simulink model "LM_TOS_0120"  (R2018b)
settings: Solver=FixedStepDiscrete  StartTime=0.0  StopTime=inf  FixedStep=0.005  RelTol=1e-3
PostLoadFcn:
  | if any(exist('dsrtsu_mdlpostloadfcn', 'file') ~= 0), dsrtsu_mdlpostloadfcn('Execute', bdroot); end
libraries: rtican x35
(part 9 of 11)

== system LM_TOS_0120/LM_TOS_MODEL/adapter2/hmi_output_adapter ==
  In1 : Inport  OutDataTypeStr=Bus: HMI_OUTPUT_ST_APT
  Bus Creator : BusCreator  Inputs=1  OutDataTypeStr=Bus: HMI_DISPLAY_ARRAY_ST  NonVirtualBus=on
  Bus Selector1 : BusSelector  OutputSignals=obj_0,obj_1,obj_2,obj_3,obj_4,obj_5,obj_6,obj_7,obj_8,obj_9,obj_10,obj_11,obj_12,obj_13,obj_14,obj_15,obj_16,obj_17,obj_18,obj_19,obj_20,obj_21,obj_22,obj_23,obj_24,obj_25,obj_26,obj_27,obj_28,obj_29,obj_30,obj_31
  Vector Concatenate : Concatenate  NumInputs=32
  Out1 : Outport  OutDataTypeStr=Bus: HMI_DISPLAY_ARRAY_ST
  wires:
  Vector Concatenate/1 -> Bus Creator/1
  In1/1 -> Bus Selector1/1
  Bus Creator/1 -> Out1/1
  Bus Selector1/9 -> Vector Concatenate/9  "<obj_8>"
  Bus Selector1/1 -> Vector Concatenate/1  "<obj_0>"
  Bus Selector1/2 -> Vector Concatenate/2  "<obj_1>"
  Bus Selector1/3 -> Vector Concatenate/3  "<obj_2>"
  Bus Selector1/4 -> Vector Concatenate/4  "<obj_3>"
  Bus Selector1/5 -> Vector Concatenate/5  "<obj_4>"
  Bus Selector1/6 -> Vector Concatenate/6  "<obj_5>"
  Bus Selector1/7 -> Vector Concatenate/7  "<obj_6>"
  Bus Selector1/8 -> Vector Concatenate/8  "<obj_7>"
  Bus Selector1/10 -> Vector Concatenate/10  "<obj_9>"
  Bus Selector1/11 -> Vector Concatenate/11  "<obj_10>"
  Bus Selector1/12 -> Vector Concatenate/12  "<obj_11>"
  Bus Selector1/13 -> Vector Concatenate/13  "<obj_12>"
  Bus Selector1/14 -> Vector Concatenate/14  "<obj_13>"
  Bus Selector1/15 -> Vector Concatenate/15  "<obj_14>"
  Bus Selector1/16 -> Vector Concatenate/16  "<obj_15>"
  Bus Selector1/17 -> Vector Concatenate/17  "<obj_16>"
  Bus Selector1/18 -> Vector Concatenate/18  "<obj_17>"
  Bus Selector1/19 -> Vector Concatenate/19  "<obj_18>"
  Bus Selector1/20 -> Vector Concatenate/20  "<obj_19>"
  Bus Selector1/21 -> Vector Concatenate/21  "<obj_20>"
  Bus Selector1/22 -> Vector Concatenate/22  "<obj_21>"
  Bus Selector1/23 -> Vector Concatenate/23  "<obj_22>"
  Bus Selector1/24 -> Vector Concatenate/24  "<obj_23>"
  Bus Selector1/25 -> Vector Concatenate/25  "<obj_24>"
  Bus Selector1/26 -> Vector Concatenate/26  "<obj_25>"
  Bus Selector1/27 -> Vector Concatenate/27  "<obj_26>"
  Bus Selector1/28 -> Vector Concatenate/28  "<obj_27>"
  Bus Selector1/29 -> Vector Concatenate/29  "<obj_28>"
  Bus Selector1/30 -> Vector Concatenate/30  "<obj_29>"
  Bus Selector1/31 -> Vector Concatenate/31  "<obj_30>"
  Bus Selector1/32 -> Vector Concatenate/32  "<obj_31>"

== system LM_TOS_0120/RTI Data/RTI Data Store/RTI Data Store ==
  RTI Data Store : Subsystem  mask(RTI_DATA_STORE){}
      mask help:
      | RTI Data Store Block. This block is used by RTI to store internal model dependent data. Deleting this block will result in data loss.
      |
      | NEVER DELETE, COPY, OR MODIFY THIS BLOCK!
      mask Help:
      | RTI Data Store Block. This block is used by RTI to store internal model dependent data. Deleting this block will result in data loss.
      | 
      | NEVER DELETE, COPY, OR MODIFY THIS BLOCK!
      mask Display: text(0.5, 0.5, ' ', 'HorizontalAlignment', 'center');

== system LM_TOS_0120/LM_TOS_MODEL/adapter2/HWA_TAR_OBJ_ADP/Subsystem0 ==
  <target_object_adapter> : Inport
  Bus Creator1 : BusCreator  Inputs=9  OutDataTypeStr=Bus: TARGETOBJECT  NonVirtualBus=on
  Bus Selector4 : BusSelector  OutputSignals=dis2EgoLaneCenter,TTC_f,ID_un8,Index_un8,probWithinLane_arr_f_0,probWithinLane_arr_f_1,probWithinLane_arr_f_2,probWithinLane_arr_f_3,probWithinLane_arr_f_4,probCutIn_f,probCutOut_f,overlap_f,trackingTimeWithinLane_f
  Vector Concatenate : Concatenate  NumInputs=5
  TARGRTOBJECTS_ST : Outport  OutDataTypeStr=Bus: TARGETOBJECT
  wires:
  Bus Selector4/8 -> Vector Concatenate/4  "<probWithinLane_arr_f_3>"
  Bus Selector4/11 -> Bus Creator1/7  "<probCutOut_f>"
  Bus Selector4/10 -> Bus Creator1/6  "<probCutIn_f>"
  Bus Selector4/12 -> Bus Creator1/8  "<overlap_f>"
  Bus Selector4/9 -> Vector Concatenate/5  "<probWithinLane_arr_f_4>"
  Bus Selector4/2 -> Bus Creator1/2  "<TTC_f>"
  Bus Selector4/5 -> Vector Concatenate/1  "<probWithinLane_arr_f_0>"
  <target_object_adapter>/1 -> Bus Selector4/1
  Bus Selector4/6 -> Vector Concatenate/2  "<probWithinLane_arr_f_1>"
  Bus Selector4/13 -> Bus Creator1/9  "<trackingTimeWithinLane_f>"
  Bus Selector4/1 -> Bus Creator1/1  "<dis2EgoLaneCenter>"
  Bus Selector4/7 -> Vector Concatenate/3  "<probWithinLane_arr_f_2>"
  Vector Concatenate/1 -> Bus Creator1/5
  Bus Selector4/3 -> Bus Creator1/3  "<ID_un8>"
  Bus Creator1/1 -> TARGRTOBJECTS_ST/1
  Bus Selector4/4 -> Bus Creator1/4  "<Index_un8>"

== system LM_TOS_0120/LM_TOS_MODEL/adapter2/HWA_TAR_OBJ_ADP/Subsystem1 ==
  <target_object_adapter> : Inport
  Bus Creator1 : BusCreator  Inputs=9  OutDataTypeStr=Bus: TARGETOBJECT  NonVirtualBus=on
  Bus Selector4 : BusSelector  OutputSignals=dis2EgoLaneCenter,TTC_f,ID_un8,Index_un8,probWithinLane_arr_f_0,probWithinLane_arr_f_1,probWithinLane_arr_f_2,probWithinLane_arr_f_3,probWithinLane_arr_f_4,probCutIn_f,probCutOut_f,overlap_f,trackingTimeWithinLane_f
  Vector Concatenate : Concatenate  NumInputs=5
  TARGRTOBJECTS_ST : Outport  OutDataTypeStr=Bus: TARGETOBJECT
  wires:
  Bus Selector4/4 -> Bus Creator1/4  "<Index_un8>"
  Bus Creator1/1 -> TARGRTOBJECTS_ST/1
  Bus Selector4/3 -> Bus Creator1/3  "<ID_un8>"
  Vector Concatenate/1 -> Bus Creator1/5
  Bus Selector4/7 -> Vector Concatenate/3  "<probWithinLane_arr_f_2>"
  Bus Selector4/1 -> Bus Creator1/1  "<dis2EgoLaneCenter>"
  Bus Selector4/13 -> Bus Creator1/9  "<trackingTimeWithinLane_f>"
  Bus Selector4/6 -> Vector Concatenate/2  "<probWithinLane_arr_f_1>"
  <target_object_adapter>/1 -> Bus Selector4/1
  Bus Selector4/5 -> Vector Concatenate/1  "<probWithinLane_arr_f_0>"
  Bus Selector4/2 -> Bus Creator1/2  "<TTC_f>"
  Bus Selector4/9 -> Vector Concatenate/5  "<probWithinLane_arr_f_4>"
  Bus Selector4/12 -> Bus Creator1/8  "<overlap_f>"
  Bus Selector4/10 -> Bus Creator1/6  "<probCutIn_f>"
  Bus Selector4/11 -> Bus Creator1/7  "<probCutOut_f>"
  Bus Selector4/8 -> Vector Concatenate/4  "<probWithinLane_arr_f_3>"

== system LM_TOS_0120/LM_TOS_MODEL/adapter2/HWA_TAR_OBJ_ADP/Subsystem10 ==
  <target_object_adapter> : Inport
  Bus Creator1 : BusCreator  Inputs=9  OutDataTypeStr=Bus: TARGETOBJECT  NonVirtualBus=on
  Bus Selector4 : BusSelector  OutputSignals=dis2EgoLaneCenter,TTC_f,ID_un8,Index_un8,probWithinLane_arr_f_0,probWithinLane_arr_f_1,probWithinLane_arr_f_2,probWithinLane_arr_f_3,probWithinLane_arr_f_4,probCutIn_f,probCutOut_f,overlap_f,trackingTimeWithinLane_f
  Vector Concatenate : Concatenate  NumInputs=5
  TARGRTOBJECTS_ST : Outport  OutDataTypeStr=Bus: TARGETOBJECT
  wires:
  Bus Selector4/8 -> Vector Concatenate/4  "<probWithinLane_arr_f_3>"
  Bus Selector4/11 -> Bus Creator1/7  "<probCutOut_f>"
  Bus Selector4/10 -> Bus Creator1/6  "<probCutIn_f>"
  Bus Selector4/12 -> Bus Creator1/8  "<overlap_f>"
  Bus Selector4/9 -> Vector Concatenate/5  "<probWithinLane_arr_f_4>"
  Bus Selector4/2 -> Bus Creator1/2  "<TTC_f>"
  Bus Selector4/5 -> Vector Concatenate/1  "<probWithinLane_arr_f_0>"
  <target_object_adapter>/1 -> Bus Selector4/1
  Bus Selector4/6 -> Vector Concatenate/2  "<probWithinLane_arr_f_1>"
  Bus Selector4/13 -> Bus Creator1/9  "<trackingTimeWithinLane_f>"
  Bus Selector4/1 -> Bus Creator1/1  "<dis2EgoLaneCenter>"
  Bus Selector4/7 -> Vector Concatenate/3  "<probWithinLane_arr_f_2>"
  Vector Concatenate/1 -> Bus Creator1/5
  Bus Selector4/3 -> Bus Creator1/3  "<ID_un8>"
  Bus Creator1/1 -> TARGRTOBJECTS_ST/1
  Bus Selector4/4 -> Bus Creator1/4  "<Index_un8>"

== system LM_TOS_0120/LM_TOS_MODEL/adapter2/HWA_TAR_OBJ_ADP/Subsystem11 ==
  <target_object_adapter> : Inport
  Bus Creator1 : BusCreator  Inputs=9  OutDataTypeStr=Bus: TARGETOBJECT  NonVirtualBus=on
  Bus Selector4 : BusSelector  OutputSignals=dis2EgoLaneCenter,TTC_f,ID_un8,Index_un8,probWithinLane_arr_f_0,probWithinLane_arr_f_1,probWithinLane_arr_f_2,probWithinLane_arr_f_3,probWithinLane_arr_f_4,probCutIn_f,probCutOut_f,overlap_f,trackingTimeWithinLane_f
  Vector Concatenate : Concatenate  NumInputs=5
  TARGRTOBJECTS_ST : Outport  OutDataTypeStr=Bus: TARGETOBJECT
  wires:
  Bus Selector4/4 -> Bus Creator1/4  "<Index_un8>"
  Bus Creator1/1 -> TARGRTOBJECTS_ST/1
  Bus Selector4/3 -> Bus Creator1/3  "<ID_un8>"
  Vector Concatenate/1 -> Bus Creator1/5
  Bus Selector4/7 -> Vector Concatenate/3  "<probWithinLane_arr_f_2>"
  Bus Selector4/1 -> Bus Creator1/1  "<dis2EgoLaneCenter>"
  Bus Selector4/13 -> Bus Creator1/9  "<trackingTimeWithinLane_f>"
  Bus Selector4/6 -> Vector Concatenate/2  "<probWithinLane_arr_f_1>"
  <target_object_adapter>/1 -> Bus Selector4/1
  Bus Selector4/5 -> Vector Concatenate/1  "<probWithinLane_arr_f_0>"
  Bus Selector4/2 -> Bus Creator1/2  "<TTC_f>"
  Bus Selector4/9 -> Vector Concatenate/5  "<probWithinLane_arr_f_4>"
  Bus Selector4/12 -> Bus Creator1/8  "<overlap_f>"
  Bus Selector4/10 -> Bus Creator1/6  "<probCutIn_f>"
  Bus Selector4/11 -> Bus Creator1/7  "<probCutOut_f>"
  Bus Selector4/8 -> Vector Concatenate/4  "<probWithinLane_arr_f_3>"

== system LM_TOS_0120/LM_TOS_MODEL/adapter2/HWA_TAR_OBJ_ADP/Subsystem2 ==
  <target_object_adapter> : Inport
  Bus Creator1 : BusCreator  Inputs=9  OutDataTypeStr=Bus: TARGETOBJECT  NonVirtualBus=on
  Bus Selector4 : BusSelector  OutputSignals=dis2EgoLaneCenter,TTC_f,ID_un8,Index_un8,probWithinLane_arr_f_0,probWithinLane_arr_f_1,probWithinLane_arr_f_2,probWithinLane_arr_f_3,probWithinLane_arr_f_4,probCutIn_f,probCutOut_f,overlap_f,trackingTimeWithinLane_f
  Vector Concatenate : Concatenate  NumInputs=5
  TARGRTOBJECTS_ST : Outport  OutDataTypeStr=Bus: TARGETOBJECT
  wires:
  Bus Selector4/8 -> Vector Concatenate/4  "<probWithinLane_arr_f_3>"
  Bus Selector4/11 -> Bus Creator1/7  "<probCutOut_f>"
  Bus Selector4/10 -> Bus Creator1/6  "<probCutIn_f>"
  Bus Selector4/12 -> Bus Creator1/8  "<overlap_f>"
  Bus Selector4/9 -> Vector Concatenate/5  "<probWithinLane_arr_f_4>"
  Bus Selector4/2 -> Bus Creator1/2  "<TTC_f>"
  Bus Selector4/5 -> Vector Concatenate/1  "<probWithinLane_arr_f_0>"
  <target_object_adapter>/1 -> Bus Selector4/1
  Bus Selector4/6 -> Vector Concatenate/2  "<probWithinLane_arr_f_1>"
  Bus Selector4/13 -> Bus Creator1/9  "<trackingTimeWithinLane_f>"
  Bus Selector4/1 -> Bus Creator1/1  "<dis2EgoLaneCenter>"
  Bus Selector4/7 -> Vector Concatenate/3  "<probWithinLane_arr_f_2>"
  Vector Concatenate/1 -> Bus Creator1/5
  Bus Selector4/3 -> Bus Creator1/3  "<ID_un8>"
  Bus Creator1/1 -> TARGRTOBJECTS_ST/1
  Bus Selector4/4 -> Bus Creator1/4  "<Index_un8>"

== system LM_TOS_0120/LM_TOS_MODEL/adapter2/HWA_TAR_OBJ_ADP/Subsystem3 ==
  <target_object_adapter> : Inport
  Bus Creator1 : BusCreator  Inputs=9  OutDataTypeStr=Bus: TARGETOBJECT  NonVirtualBus=on
  Bus Selector4 : BusSelector  OutputSignals=dis2EgoLaneCenter,TTC_f,ID_un8,Index_un8,probWithinLane_arr_f_0,probWithinLane_arr_f_1,probWithinLane_arr_f_2,probWithinLane_arr_f_3,probWithinLane_arr_f_4,probCutIn_f,probCutOut_f,overlap_f,trackingTimeWithinLane_f
  Vector Concatenate : Concatenate  NumInputs=5
  TARGRTOBJECTS_ST : Outport  OutDataTypeStr=Bus: TARGETOBJECT
  wires:
  Bus Selector4/4 -> Bus Creator1/4  "<Index_un8>"
  Bus Creator1/1 -> TARGRTOBJECTS_ST/1
  Bus Selector4/3 -> Bus Creator1/3  "<ID_un8>"
  Vector Concatenate/1 -> Bus Creator1/5
  Bus Selector4/7 -> Vector Concatenate/3  "<probWithinLane_arr_f_2>"
  Bus Selector4/1 -> Bus Creator1/1  "<dis2EgoLaneCenter>"
  Bus Selector4/13 -> Bus Creator1/9  "<trackingTimeWithinLane_f>"
  Bus Selector4/6 -> Vector Concatenate/2  "<probWithinLane_arr_f_1>"
  <target_object_adapter>/1 -> Bus Selector4/1
  Bus Selector4/5 -> Vector Concatenate/1  "<probWithinLane_arr_f_0>"
  Bus Selector4/2 -> Bus Creator1/2  "<TTC_f>"
  Bus Selector4/9 -> Vector Concatenate/5  "<probWithinLane_arr_f_4>"
  Bus Selector4/12 -> Bus Creator1/8  "<overlap_f>"
  Bus Selector4/10 -> Bus Creator1/6  "<probCutIn_f>"
  Bus Selector4/11 -> Bus Creator1/7  "<probCutOut_f>"
  Bus Selector4/8 -> Vector Concatenate/4  "<probWithinLane_arr_f_3>"

== system LM_TOS_0120/LM_TOS_MODEL/adapter2/HWA_TAR_OBJ_ADP/Subsystem4 ==
  <target_object_adapter> : Inport
  Bus Creator1 : BusCreator  Inputs=9  OutDataTypeStr=Bus: TARGETOBJECT  NonVirtualBus=on
  Bus Selector4 : BusSelector  OutputSignals=dis2EgoLaneCenter,TTC_f,ID_un8,Index_un8,probWithinLane_arr_f_0,probWithinLane_arr_f_1,probWithinLane_arr_f_2,probWithinLane_arr_f_3,probWithinLane_arr_f_4,probCutIn_f,probCutOut_f,overlap_f,trackingTimeWithinLane_f
  Vector Concatenate : Concatenate  NumInputs=5
  TARGRTOBJECTS_ST : Outport  OutDataTypeStr=Bus: TARGETOBJECT
  wires:
  Bus Selector4/8 -> Vector Concatenate/4  "<probWithinLane_arr_f_3>"
  Bus Selector4/11 -> Bus Creator1/7  "<probCutOut_f>"
  Bus Selector4/10 -> Bus Creator1/6  "<probCutIn_f>"
  Bus Selector4/12 -> Bus Creator1/8  "<overlap_f>"
  Bus Selector4/9 -> Vector Concatenate/5  "<probWithinLane_arr_f_4>"
  Bus Selector4/2 -> Bus Creator1/2  "<TTC_f>"
  Bus Selector4/5 -> Vector Concatenate/1  "<probWithinLane_arr_f_0>"
  <target_object_adapter>/1 -> Bus Selector4/1
  Bus Selector4/6 -> Vector Concatenate/2  "<probWithinLane_arr_f_1>"
  Bus Selector4/13 -> Bus Creator1/9  "<trackingTimeWithinLane_f>"
  Bus Selector4/1 -> Bus Creator1/1  "<dis2EgoLaneCenter>"
  Bus Selector4/7 -> Vector Concatenate/3  "<probWithinLane_arr_f_2>"
  Vector Concatenate/1 -> Bus Creator1/5
  Bus Selector4/3 -> Bus Creator1/3  "<ID_un8>"
  Bus Creator1/1 -> TARGRTOBJECTS_ST/1
  Bus Selector4/4 -> Bus Creator1/4  "<Index_un8>"

== system LM_TOS_0120/LM_TOS_MODEL/adapter2/HWA_TAR_OBJ_ADP/Subsystem5 ==
  <target_object_adapter> : Inport
  Bus Creator1 : BusCreator  Inputs=9  OutDataTypeStr=Bus: TARGETOBJECT  NonVirtualBus=on
  Bus Selector4 : BusSelector  OutputSignals=dis2EgoLaneCenter,TTC_f,ID_un8,Index_un8,probWithinLane_arr_f_0,probWithinLane_arr_f_1,probWithinLane_arr_f_2,probWithinLane_arr_f_3,probWithinLane_arr_f_4,probCutIn_f,probCutOut_f,overlap_f,trackingTimeWithinLane_f
  Vector Concatenate : Concatenate  NumInputs=5
  TARGRTOBJECTS_ST : Outport  OutDataTypeStr=Bus: TARGETOBJECT
  wires:
  Bus Selector4/4 -> Bus Creator1/4  "<Index_un8>"
  Bus Creator1/1 -> TARGRTOBJECTS_ST/1
  Bus Selector4/3 -> Bus Creator1/3  "<ID_un8>"
  Vector Concatenate/1 -> Bus Creator1/5
  Bus Selector4/7 -> Vector Concatenate/3  "<probWithinLane_arr_f_2>"
  Bus Selector4/1 -> Bus Creator1/1  "<dis2EgoLaneCenter>"
  Bus Selector4/13 -> Bus Creator1/9  "<trackingTimeWithinLane_f>"
  Bus Selector4/6 -> Vector Concatenate/2  "<probWithinLane_arr_f_1>"
  <target_object_adapter>/1 -> Bus Selector4/1
  Bus Selector4/5 -> Vector Concatenate/1  "<probWithinLane_arr_f_0>"
  Bus Selector4/2 -> Bus Creator1/2  "<TTC_f>"
  Bus Selector4/9 -> Vector Concatenate/5  "<probWithinLane_arr_f_4>"
  Bus Selector4/12 -> Bus Creator1/8  "<overlap_f>"
  Bus Selector4/10 -> Bus Creator1/6  "<probCutIn_f>"
  Bus Selector4/11 -> Bus Creator1/7  "<probCutOut_f>"
  Bus Selector4/8 -> Vector Concatenate/4  "<probWithinLane_arr_f_3>"

== system LM_TOS_0120/LM_TOS_MODEL/adapter2/HWA_TAR_OBJ_ADP/Subsystem6 ==
  <target_object_adapter> : Inport
  Bus Creator1 : BusCreator  Inputs=9  OutDataTypeStr=Bus: TARGETOBJECT  NonVirtualBus=on
  Bus Selector4 : BusSelector  OutputSignals=dis2EgoLaneCenter,TTC_f,ID_un8,Index_un8,probWithinLane_arr_f_0,probWithinLane_arr_f_1,probWithinLane_arr_f_2,probWithinLane_arr_f_3,probWithinLane_arr_f_4,probCutIn_f,probCutOut_f,overlap_f,trackingTimeWithinLane_f
  Vector Concatenate : Concatenate  NumInputs=5
  TARGRTOBJECTS_ST : Outport  OutDataTypeStr=Bus: TARGETOBJECT
  wires:
  Bus Selector4/8 -> Vector Concatenate/4  "<probWithinLane_arr_f_3>"
  Bus Selector4/11 -> Bus Creator1/7  "<probCutOut_f>"
  Bus Selector4/10 -> Bus Creator1/6  "<probCutIn_f>"
  Bus Selector4/12 -> Bus Creator1/8  "<overlap_f>"
  Bus Selector4/9 -> Vector Concatenate/5  "<probWithinLane_arr_f_4>"
  Bus Selector4/2 -> Bus Creator1/2  "<TTC_f>"
  Bus Selector4/5 -> Vector Concatenate/1  "<probWithinLane_arr_f_0>"
  <target_object_adapter>/1 -> Bus Selector4/1
  Bus Selector4/6 -> Vector Concatenate/2  "<probWithinLane_arr_f_1>"
  Bus Selector4/13 -> Bus Creator1/9  "<trackingTimeWithinLane_f>"
  Bus Selector4/1 -> Bus Creator1/1  "<dis2EgoLaneCenter>"
  Bus Selector4/7 -> Vector Concatenate/3  "<probWithinLane_arr_f_2>"
  Vector Concatenate/1 -> Bus Creator1/5
  Bus Selector4/3 -> Bus Creator1/3  "<ID_un8>"
  Bus Creator1/1 -> TARGRTOBJECTS_ST/1
  Bus Selector4/4 -> Bus Creator1/4  "<Index_un8>"

== system LM_TOS_0120/LM_TOS_MODEL/adapter2/HWA_TAR_OBJ_ADP/Subsystem7 ==
  <target_object_adapter> : Inport
  Bus Creator1 : BusCreator  Inputs=9  OutDataTypeStr=Bus: TARGETOBJECT  NonVirtualBus=on
  Bus Selector4 : BusSelector  OutputSignals=dis2EgoLaneCenter,TTC_f,ID_un8,Index_un8,probWithinLane_arr_f_0,probWithinLane_arr_f_1,probWithinLane_arr_f_2,probWithinLane_arr_f_3,probWithinLane_arr_f_4,probCutIn_f,probCutOut_f,overlap_f,trackingTimeWithinLane_f
  Vector Concatenate : Concatenate  NumInputs=5
  TARGRTOBJECTS_ST : Outport  OutDataTypeStr=Bus: TARGETOBJECT
  wires:
  Bus Selector4/4 -> Bus Creator1/4  "<Index_un8>"
  Bus Creator1/1 -> TARGRTOBJECTS_ST/1
  Bus Selector4/3 -> Bus Creator1/3  "<ID_un8>"
  Vector Concatenate/1 -> Bus Creator1/5
  Bus Selector4/7 -> Vector Concatenate/3  "<probWithinLane_arr_f_2>"
  Bus Selector4/1 -> Bus Creator1/1  "<dis2EgoLaneCenter>"
  Bus Selector4/13 -> Bus Creator1/9  "<trackingTimeWithinLane_f>"
  Bus Selector4/6 -> Vector Concatenate/2  "<probWithinLane_arr_f_1>"
  <target_object_adapter>/1 -> Bus Selector4/1
  Bus Selector4/5 -> Vector Concatenate/1  "<probWithinLane_arr_f_0>"
  Bus Selector4/2 -> Bus Creator1/2  "<TTC_f>"
  Bus Selector4/9 -> Vector Concatenate/5  "<probWithinLane_arr_f_4>"
  Bus Selector4/12 -> Bus Creator1/8  "<overlap_f>"
  Bus Selector4/10 -> Bus Creator1/6  "<probCutIn_f>"
  Bus Selector4/11 -> Bus Creator1/7  "<probCutOut_f>"
  Bus Selector4/8 -> Vector Concatenate/4  "<probWithinLane_arr_f_3>"

== system LM_TOS_0120/LM_TOS_MODEL/adapter2/HWA_TAR_OBJ_ADP/Subsystem8 ==
  <target_object_adapter> : Inport
  Bus Creator1 : BusCreator  Inputs=9  OutDataTypeStr=Bus: TARGETOBJECT  NonVirtualBus=on
  Bus Selector4 : BusSelector  OutputSignals=dis2EgoLaneCenter,TTC_f,ID_un8,Index_un8,probWithinLane_arr_f_0,probWithinLane_arr_f_1,probWithinLane_arr_f_2,probWithinLane_arr_f_3,probWithinLane_arr_f_4,probCutIn_f,probCutOut_f,overlap_f,trackingTimeWithinLane_f
  Vector Concatenate : Concatenate  NumInputs=5
  TARGRTOBJECTS_ST : Outport  OutDataTypeStr=Bus: TARGETOBJECT
  wires:
  Bus Selector4/8 -> Vector Concatenate/4  "<probWithinLane_arr_f_3>"
  Bus Selector4/11 -> Bus Creator1/7  "<probCutOut_f>"
  Bus Selector4/10 -> Bus Creator1/6  "<probCutIn_f>"
  Bus Selector4/12 -> Bus Creator1/8  "<overlap_f>"
  Bus Selector4/9 -> Vector Concatenate/5  "<probWithinLane_arr_f_4>"
  Bus Selector4/2 -> Bus Creator1/2  "<TTC_f>"
  Bus Selector4/5 -> Vector Concatenate/1  "<probWithinLane_arr_f_0>"
  <target_object_adapter>/1 -> Bus Selector4/1
  Bus Selector4/6 -> Vector Concatenate/2  "<probWithinLane_arr_f_1>"
  Bus Selector4/13 -> Bus Creator1/9  "<trackingTimeWithinLane_f>"
  Bus Selector4/1 -> Bus Creator1/1  "<dis2EgoLaneCenter>"
  Bus Selector4/7 -> Vector Concatenate/3  "<probWithinLane_arr_f_2>"
  Vector Concatenate/1 -> Bus Creator1/5
  Bus Selector4/3 -> Bus Creator1/3  "<ID_un8>"
  Bus Creator1/1 -> TARGRTOBJECTS_ST/1
  Bus Selector4/4 -> Bus Creator1/4  "<Index_un8>"

== system LM_TOS_0120/LM_TOS_MODEL/adapter2/HWA_TAR_OBJ_ADP/Subsystem9 ==
  <target_object_adapter> : Inport
  Bus Creator1 : BusCreator  Inputs=9  OutDataTypeStr=Bus: TARGETOBJECT  NonVirtualBus=on
  Bus Selector4 : BusSelector  OutputSignals=dis2EgoLaneCenter,TTC_f,ID_un8,Index_un8,probWithinLane_arr_f_0,probWithinLane_arr_f_1,probWithinLane_arr_f_2,probWithinLane_arr_f_3,probWithinLane_arr_f_4,probCutIn_f,probCutOut_f,overlap_f,trackingTimeWithinLane_f
  Vector Concatenate : Concatenate  NumInputs=5
  TARGRTOBJECTS_ST : Outport  OutDataTypeStr=Bus: TARGETOBJECT
  wires:
  Bus Selector4/4 -> Bus Creator1/4  "<Index_un8>"
  Bus Creator1/1 -> TARGRTOBJECTS_ST/1
  Bus Selector4/3 -> Bus Creator1/3  "<ID_un8>"
  Vector Concatenate/1 -> Bus Creator1/5
  Bus Selector4/7 -> Vector Concatenate/3  "<probWithinLane_arr_f_2>"
  Bus Selector4/1 -> Bus Creator1/1  "<dis2EgoLaneCenter>"
  Bus Selector4/13 -> Bus Creator1/9  "<trackingTimeWithinLane_f>"
  Bus Selector4/6 -> Vector Concatenate/2  "<probWithinLane_arr_f_1>"
  <target_object_adapter>/1 -> Bus Selector4/1
  Bus Selector4/5 -> Vector Concatenate/1  "<probWithinLane_arr_f_0>"
  Bus Selector4/2 -> Bus Creator1/2  "<TTC_f>"
  Bus Selector4/9 -> Vector Concatenate/5  "<probWithinLane_arr_f_4>"
  Bus Selector4/12 -> Bus Creator1/8  "<overlap_f>"
  Bus Selector4/10 -> Bus Creator1/6  "<probCutIn_f>"
  Bus Selector4/11 -> Bus Creator1/7  "<probCutOut_f>"
  Bus Selector4/8 -> Vector Concatenate/4  "<probWithinLane_arr_f_3>"

== system LM_TOS_0120/LM_TOS_MODEL/adapter2/Lane_0/Subsystem ==
  <LANE_0_TARGETOBJECT_0_ST> : Inport
  Bus Creator1 : BusCreator  Inputs=9  OutDataTypeStr=Bus: TARGETOBJECT  NonVirtualBus=on
  Bus Selector4 : BusSelector  OutputSignals=dis2EgoLaneCenter,TTC_f,ID_un8,Index_un8,probWithinLane_arr_f_0,probWithinLane_arr_f_1,probWithinLane_arr_f_2,probWithinLane_arr_f_3,probWithinLane_arr_f_4,probCutIn_f,probCutOut_f,overlap_f,trackingTimeWithinLane_f
  Vector Concatenate : Concatenate  NumInputs=5
  TARGRTOBJECTS_ST : Outport  OutDataTypeStr=Bus: TARGETOBJECT
  wires:
  Bus Selector4/4 -> Bus Creator1/4  "<Index_un8>"
  Bus Creator1/1 -> TARGRTOBJECTS_ST/1
  Bus Selector4/3 -> Bus Creator1/3  "<ID_un8>"
  Vector Concatenate/1 -> Bus Creator1/5
  Bus Selector4/7 -> Vector Concatenate/3  "<probWithinLane_arr_f_2>"
  Bus Selector4/1 -> Bus Creator1/1  "<dis2EgoLaneCenter>"
  Bus Selector4/13 -> Bus Creator1/9  "<trackingTimeWithinLane_f>"
  Bus Selector4/6 -> Vector Concatenate/2  "<probWithinLane_arr_f_1>"
  <LANE_0_TARGETOBJECT_0_ST>/1 -> Bus Selector4/1
  Bus Selector4/5 -> Vector Concatenate/1  "<probWithinLane_arr_f_0>"
  Bus Selector4/2 -> Bus Creator1/2  "<TTC_f>"
  Bus Selector4/9 -> Vector Concatenate/5  "<probWithinLane_arr_f_4>"
  Bus Selector4/12 -> Bus Creator1/8  "<overlap_f>"
  Bus Selector4/10 -> Bus Creator1/6  "<probCutIn_f>"
  Bus Selector4/11 -> Bus Creator1/7  "<probCutOut_f>"
  Bus Selector4/8 -> Vector Concatenate/4  "<probWithinLane_arr_f_3>"

== system LM_TOS_0120/LM_TOS_MODEL/adapter2/Lane_0/Subsystem1 ==
  <LANE_0_TARGETOBJECT_0_ST> : Inport
  Bus Creator1 : BusCreator  Inputs=9  OutDataTypeStr=Bus: TARGETOBJECT  NonVirtualBus=on
  Bus Selector4 : BusSelector  OutputSignals=dis2EgoLaneCenter,TTC_f,ID_un8,Index_un8,probWithinLane_arr_f_0,probWithinLane_arr_f_1,probWithinLane_arr_f_2,probWithinLane_arr_f_3,probWithinLane_arr_f_4,probCutIn_f,probCutOut_f,overlap_f,trackingTimeWithinLane_f
  Vector Concatenate : Concatenate  NumInputs=5
  TARGRTOBJECTS_ST : Outport  OutDataTypeStr=Bus: TARGETOBJECT
  wires:
  Bus Selector4/8 -> Vector Concatenate/4  "<probWithinLane_arr_f_3>"
  Bus Selector4/11 -> Bus Creator1/7  "<probCutOut_f>"
  Bus Selector4/10 -> Bus Creator1/6  "<probCutIn_f>"
  Bus Selector4/12 -> Bus Creator1/8  "<overlap_f>"
  Bus Selector4/9 -> Vector Concatenate/5  "<probWithinLane_arr_f_4>"
  Bus Selector4/2 -> Bus Creator1/2  "<TTC_f>"
  Bus Selector4/5 -> Vector Concatenate/1  "<probWithinLane_arr_f_0>"
  <LANE_0_TARGETOBJECT_0_ST>/1 -> Bus Selector4/1
  Bus Selector4/6 -> Vector Concatenate/2  "<probWithinLane_arr_f_1>"
  Bus Selector4/13 -> Bus Creator1/9  "<trackingTimeWithinLane_f>"
  Bus Selector4/1 -> Bus Creator1/1  "<dis2EgoLaneCenter>"
  Bus Selector4/7 -> Vector Concatenate/3  "<probWithinLane_arr_f_2>"
  Vector Concatenate/1 -> Bus Creator1/5
  Bus Selector4/3 -> Bus Creator1/3  "<ID_un8>"
  Bus Creator1/1 -> TARGRTOBJECTS_ST/1
  Bus Selector4/4 -> Bus Creator1/4  "<Index_un8>"

== system LM_TOS_0120/LM_TOS_MODEL/adapter2/Lane_0/Subsystem10 ==
  <LANE_0_TARGETOBJECT_0_ST> : Inport
  Bus Creator1 : BusCreator  Inputs=7  OutDataTypeStr=Bus: SEGMENT  NonVirtualBus=on
  Bus Selector4 : BusSelector  OutputSignals=coef_arr_f_0,coef_arr_f_1,coef_arr_f_2,coef_arr_f_3,dlowerLimit_f,dupperLimit_f,numOfSegment_un8,available_b,detectedByVideo_b,quality_f
  Vector Concatenate : Concatenate  NumInputs=4
  SEGMENT_ST : Outport  OutDataTypeStr=Bus: SEGMENT
  wires:
  Bus Creator1/1 -> SEGMENT_ST/1
  <LANE_0_TARGETOBJECT_0_ST>/1 -> Bus Selector4/1
  Bus Selector4/2 -> Vector Concatenate/2  "<coef_arr_f_1>"
  Bus Selector4/1 -> Vector Concatenate/1  "<coef_arr_f_0>"
  Bus Selector4/3 -> Vector Concatenate/3  "<coef_arr_f_2>"
  Bus Selector4/4 -> Vector Concatenate/4  "<coef_arr_f_3>"
  Vector Concatenate/1 -> Bus Creator1/1
  Bus Selector4/5 -> Bus Creator1/2  "<dlowerLimit_f>"
  Bus Selector4/10 -> Bus Creator1/7  "<quality_f>"
  Bus Selector4/9 -> Bus Creator1/6  "<detectedByVideo_b>"
  Bus Selector4/8 -> Bus Creator1/5  "<available_b>"
  Bus Selector4/7 -> Bus Creator1/4  "<numOfSegment_un8>"
  Bus Selector4/6 -> Bus Creator1/3  "<dupperLimit_f>"

== system LM_TOS_0120/LM_TOS_MODEL/adapter2/Lane_0/Subsystem11 ==
  <LANE_0_TARGETOBJECT_0_ST> : Inport
  Bus Creator1 : BusCreator  Inputs=7  OutDataTypeStr=Bus: SEGMENT  NonVirtualBus=on
  Bus Selector4 : BusSelector  OutputSignals=coef_arr_f_0,coef_arr_f_1,coef_arr_f_2,coef_arr_f_3,dlowerLimit_f,dupperLimit_f,numOfSegment_un8,available_b,detectedByVideo_b,quality_f
  Vector Concatenate : Concatenate  NumInputs=4
  SEGMENT_ST : Outport  OutDataTypeStr=Bus: SEGMENT
  wires:
  Bus Selector4/6 -> Bus Creator1/3  "<dupperLimit_f>"
  Bus Selector4/7 -> Bus Creator1/4  "<numOfSegment_un8>"
  Bus Selector4/8 -> Bus Creator1/5  "<available_b>"
  Bus Selector4/9 -> Bus Creator1/6  "<detectedByVideo_b>"
  Bus Selector4/10 -> Bus Creator1/7  "<quality_f>"
  Bus Selector4/5 -> Bus Creator1/2  "<dlowerLimit_f>"
  Vector Concatenate/1 -> Bus Creator1/1
  Bus Selector4/4 -> Vector Concatenate/4  "<coef_arr_f_3>"
  Bus Selector4/3 -> Vector Concatenate/3  "<coef_arr_f_2>"
  Bus Selector4/1 -> Vector Concatenate/1  "<coef_arr_f_0>"
  Bus Selector4/2 -> Vector Concatenate/2  "<coef_arr_f_1>"
  <LANE_0_TARGETOBJECT_0_ST>/1 -> Bus Selector4/1
  Bus Creator1/1 -> SEGMENT_ST/1

== system LM_TOS_0120/LM_TOS_MODEL/adapter2/Lane_0/Subsystem12 ==
  <LANE_0_TARGETOBJECT_0_ST> : Inport
  Bus Creator1 : BusCreator  Inputs=7  OutDataTypeStr=Bus: SEGMENT  NonVirtualBus=on
  Bus Selector4 : BusSelector  OutputSignals=coef_arr_f_0,coef_arr_f_1,coef_arr_f_2,coef_arr_f_3,dlowerLimit_f,dupperLimit_f,numOfSegment_un8,available_b,detectedByVideo_b,quality_f
  Vector Concatenate : Concatenate  NumInputs=4
  SEGMENT_ST : Outport  OutDataTypeStr=Bus: SEGMENT
  wires:
  Bus Creator1/1 -> SEGMENT_ST/1
  <LANE_0_TARGETOBJECT_0_ST>/1 -> Bus Selector4/1
  Bus Selector4/2 -> Vector Concatenate/2  "<coef_arr_f_1>"
  Bus Selector4/1 -> Vector Concatenate/1  "<coef_arr_f_0>"
  Bus Selector4/3 -> Vector Concatenate/3  "<coef_arr_f_2>"
  Bus Selector4/4 -> Vector Concatenate/4  "<coef_arr_f_3>"
  Vector Concatenate/1 -> Bus Creator1/1
  Bus Selector4/5 -> Bus Creator1/2  "<dlowerLimit_f>"
  Bus Selector4/10 -> Bus Creator1/7  "<quality_f>"
  Bus Selector4/9 -> Bus Creator1/6  "<detectedByVideo_b>"
  Bus Selector4/8 -> Bus Creator1/5  "<available_b>"
  Bus Selector4/7 -> Bus Creator1/4  "<numOfSegment_un8>"
  Bus Selector4/6 -> Bus Creator1/3  "<dupperLimit_f>"

== system LM_TOS_0120/LM_TOS_MODEL/adapter2/Lane_0/Subsystem13 ==
  <LANE_0_TARGETOBJECT_0_ST> : Inport
  Bus Creator1 : BusCreator  Inputs=7  OutDataTypeStr=Bus: SEGMENT  NonVirtualBus=on
  Bus Selector4 : BusSelector  OutputSignals=coef_arr_f_0,coef_arr_f_1,coef_arr_f_2,coef_arr_f_3,dlowerLimit_f,dupperLimit_f,numOfSegment_un8,available_b,detectedByVideo_b,quality_f
  Vector Concatenate : Concatenate  NumInputs=4
  SEGMENT_ST : Outport  OutDataTypeStr=Bus: SEGMENT
  wires:
  Bus Selector4/6 -> Bus Creator1/3  "<dupperLimit_f>"
  Bus Selector4/7 -> Bus Creator1/4  "<numOfSegment_un8>"
  Bus Selector4/8 -> Bus Creator1/5  "<available_b>"
  Bus Selector4/9 -> Bus Creator1/6  "<detectedByVideo_b>"
  Bus Selector4/10 -> Bus Creator1/7  "<quality_f>"
  Bus Selector4/5 -> Bus Creator1/2  "<dlowerLimit_f>"
  Vector Concatenate/1 -> Bus Creator1/1
  Bus Selector4/4 -> Vector Concatenate/4  "<coef_arr_f_3>"
  Bus Selector4/3 -> Vector Concatenate/3  "<coef_arr_f_2>"
  Bus Selector4/1 -> Vector Concatenate/1  "<coef_arr_f_0>"
  Bus Selector4/2 -> Vector Concatenate/2  "<coef_arr_f_1>"
  <LANE_0_TARGETOBJECT_0_ST>/1 -> Bus Selector4/1
  Bus Creator1/1 -> SEGMENT_ST/1

== system LM_TOS_0120/LM_TOS_MODEL/adapter2/Lane_0/Subsystem14 ==
  <LANE_0_TARGETOBJECT_0_ST> : Inport
  Bus Creator1 : BusCreator  Inputs=7  OutDataTypeStr=Bus: SEGMENT  NonVirtualBus=on
  Bus Selector4 : BusSelector  OutputSignals=coef_arr_f_0,coef_arr_f_1,coef_arr_f_2,coef_arr_f_3,dlowerLimit_f,dupperLimit_f,numOfSegment_un8,available_b,detectedByVideo_b,quality_f
  Vector Concatenate : Concatenate  NumInputs=4
  SEGMENT_ST : Outport  OutDataTypeStr=Bus: SEGMENT
  wires:
  Bus Creator1/1 -> SEGMENT_ST/1
  <LANE_0_TARGETOBJECT_0_ST>/1 -> Bus Selector4/1
  Bus Selector4/2 -> Vector Concatenate/2  "<coef_arr_f_1>"
  Bus Selector4/1 -> Vector Concatenate/1  "<coef_arr_f_0>"
  Bus Selector4/3 -> Vector Concatenate/3  "<coef_arr_f_2>"
  Bus Selector4/4 -> Vector Concatenate/4  "<coef_arr_f_3>"
  Vector Concatenate/1 -> Bus Creator1/1
  Bus Selector4/5 -> Bus Creator1/2  "<dlowerLimit_f>"
  Bus Selector4/10 -> Bus Creator1/7  "<quality_f>"
  Bus Selector4/9 -> Bus Creator1/6  "<detectedByVideo_b>"
  Bus Selector4/8 -> Bus Creator1/5  "<available_b>"
  Bus Selector4/7 -> Bus Creator1/4  "<numOfSegment_un8>"
  Bus Selector4/6 -> Bus Creator1/3  "<dupperLimit_f>"

== system LM_TOS_0120/LM_TOS_MODEL/adapter2/Lane_0/Subsystem15 ==
  <LANE_0_TARGETOBJECT_0_ST> : Inport
  Bus Creator1 : BusCreator  Inputs=7  OutDataTypeStr=Bus: SEGMENT  NonVirtualBus=on
  Bus Selector4 : BusSelector  OutputSignals=coef_arr_f_0,coef_arr_f_1,coef_arr_f_2,coef_arr_f_3,dlowerLimit_f,dupperLimit_f,numOfSegment_un8,available_b,detectedByVideo_b,quality_f
  Vector Concatenate : Concatenate  NumInputs=4
  SEGMENT_ST : Outport  OutDataTypeStr=Bus: SEGMENT
  wires:
  Bus Selector4/6 -> Bus Creator1/3  "<dupperLimit_f>"
  Bus Selector4/7 -> Bus Creator1/4  "<numOfSegment_un8>"
  Bus Selector4/8 -> Bus Creator1/5  "<available_b>"
  Bus Selector4/9 -> Bus Creator1/6  "<detectedByVideo_b>"
  Bus Selector4/10 -> Bus Creator1/7  "<quality_f>"
  Bus Selector4/5 -> Bus Creator1/2  "<dlowerLimit_f>"
  Vector Concatenate/1 -> Bus Creator1/1
  Bus Selector4/4 -> Vector Concatenate/4  "<coef_arr_f_3>"
  Bus Selector4/3 -> Vector Concatenate/3  "<coef_arr_f_2>"
  Bus Selector4/1 -> Vector Concatenate/1  "<coef_arr_f_0>"
  Bus Selector4/2 -> Vector Concatenate/2  "<coef_arr_f_1>"
  <LANE_0_TARGETOBJECT_0_ST>/1 -> Bus Selector4/1
  Bus Creator1/1 -> SEGMENT_ST/1

== system LM_TOS_0120/LM_TOS_MODEL/adapter2/Lane_0/Subsystem2 ==
  <LANE_0_TARGETOBJECT_0_ST> : Inport
  Bus Creator1 : BusCreator  Inputs=9  OutDataTypeStr=Bus: TARGETOBJECT  NonVirtualBus=on
  Bus Selector4 : BusSelector  OutputSignals=dis2EgoLaneCenter,TTC_f,ID_un8,Index_un8,probWithinLane_arr_f_0,probWithinLane_arr_f_1,probWithinLane_arr_f_2,probWithinLane_arr_f_3,probWithinLane_arr_f_4,probCutIn_f,probCutOut_f,overlap_f,trackingTimeWithinLane_f
  Vector Concatenate : Concatenate  NumInputs=5
  TARGRTOBJECTS_ST : Outport  OutDataTypeStr=Bus: TARGETOBJECT
  wires:
  Bus Selector4/4 -> Bus Creator1/4  "<Index_un8>"
  Bus Creator1/1 -> TARGRTOBJECTS_ST/1
  Bus Selector4/3 -> Bus Creator1/3  "<ID_un8>"
  Vector Concatenate/1 -> Bus Creator1/5
  Bus Selector4/7 -> Vector Concatenate/3  "<probWithinLane_arr_f_2>"
  Bus Selector4/1 -> Bus Creator1/1  "<dis2EgoLaneCenter>"
  Bus Selector4/13 -> Bus Creator1/9  "<trackingTimeWithinLane_f>"
  Bus Selector4/6 -> Vector Concatenate/2  "<probWithinLane_arr_f_1>"
  <LANE_0_TARGETOBJECT_0_ST>/1 -> Bus Selector4/1
  Bus Selector4/5 -> Vector Concatenate/1  "<probWithinLane_arr_f_0>"
  Bus Selector4/2 -> Bus Creator1/2  "<TTC_f>"
  Bus Selector4/9 -> Vector Concatenate/5  "<probWithinLane_arr_f_4>"
  Bus Selector4/12 -> Bus Creator1/8  "<overlap_f>"
  Bus Selector4/10 -> Bus Creator1/6  "<probCutIn_f>"
  Bus Selector4/11 -> Bus Creator1/7  "<probCutOut_f>"
  Bus Selector4/8 -> Vector Concatenate/4  "<probWithinLane_arr_f_3>"

== system LM_TOS_0120/LM_TOS_MODEL/adapter2/Lane_0/Subsystem3 ==
  <LANE_0_TARGETOBJECT_0_ST> : Inport
  Bus Creator1 : BusCreator  Inputs=9  OutDataTypeStr=Bus: TARGETOBJECT  NonVirtualBus=on
  Bus Selector4 : BusSelector  OutputSignals=dis2EgoLaneCenter,TTC_f,ID_un8,Index_un8,probWithinLane_arr_f_0,probWithinLane_arr_f_1,probWithinLane_arr_f_2,probWithinLane_arr_f_3,probWithinLane_arr_f_4,probCutIn_f,probCutOut_f,overlap_f,trackingTimeWithinLane_f
  Vector Concatenate : Concatenate  NumInputs=5
  TARGRTOBJECTS_ST : Outport  OutDataTypeStr=Bus: TARGETOBJECT
  wires:
  Bus Selector4/8 -> Vector Concatenate/4  "<probWithinLane_arr_f_3>"
  Bus Selector4/11 -> Bus Creator1/7  "<probCutOut_f>"
  Bus Selector4/10 -> Bus Creator1/6  "<probCutIn_f>"
  Bus Selector4/12 -> Bus Creator1/8  "<overlap_f>"
  Bus Selector4/9 -> Vector Concatenate/5  "<probWithinLane_arr_f_4>"
  Bus Selector4/2 -> Bus Creator1/2  "<TTC_f>"
  Bus Selector4/5 -> Vector Concatenate/1  "<probWithinLane_arr_f_0>"
  <LANE_0_TARGETOBJECT_0_ST>/1 -> Bus Selector4/1
  Bus Selector4/6 -> Vector Concatenate/2  "<probWithinLane_arr_f_1>"
  Bus Selector4/13 -> Bus Creator1/9  "<trackingTimeWithinLane_f>"
  Bus Selector4/1 -> Bus Creator1/1  "<dis2EgoLaneCenter>"
  Bus Selector4/7 -> Vector Concatenate/3  "<probWithinLane_arr_f_2>"
  Vector Concatenate/1 -> Bus Creator1/5
  Bus Selector4/3 -> Bus Creator1/3  "<ID_un8>"
  Bus Creator1/1 -> TARGRTOBJECTS_ST/1
  Bus Selector4/4 -> Bus Creator1/4  "<Index_un8>"

== system LM_TOS_0120/LM_TOS_MODEL/adapter2/Lane_0/Subsystem4 ==
  <LANE_0_TARGETOBJECT_0_ST> : Inport
  Bus Creator1 : BusCreator  Inputs=9  OutDataTypeStr=Bus: TARGETOBJECT  NonVirtualBus=on
  Bus Selector4 : BusSelector  OutputSignals=dis2EgoLaneCenter,TTC_f,ID_un8,Index_un8,probWithinLane_arr_f_0,probWithinLane_arr_f_1,probWithinLane_arr_f_2,probWithinLane_arr_f_3,probWithinLane_arr_f_4,probCutIn_f,probCutOut_f,overlap_f,trackingTimeWithinLane_f
  Vector Concatenate : Concatenate  NumInputs=5
  TARGRTOBJECTS_ST : Outport  OutDataTypeStr=Bus: TARGETOBJECT
  wires:
  Bus Selector4/4 -> Bus Creator1/4  "<Index_un8>"
  Bus Creator1/1 -> TARGRTOBJECTS_ST/1
  Bus Selector4/3 -> Bus Creator1/3  "<ID_un8>"
  Vector Concatenate/1 -> Bus Creator1/5
  Bus Selector4/7 -> Vector Concatenate/3  "<probWithinLane_arr_f_2>"
  Bus Selector4/1 -> Bus Creator1/1  "<dis2EgoLaneCenter>"
  Bus Selector4/13 -> Bus Creator1/9  "<trackingTimeWithinLane_f>"
  Bus Selector4/6 -> Vector Concatenate/2  "<probWithinLane_arr_f_1>"
  <LANE_0_TARGETOBJECT_0_ST>/1 -> Bus Selector4/1
  Bus Selector4/5 -> Vector Concatenate/1  "<probWithinLane_arr_f_0>"
  Bus Selector4/2 -> Bus Creator1/2  "<TTC_f>"
  Bus Selector4/9 -> Vector Concatenate/5  "<probWithinLane_arr_f_4>"
  Bus Selector4/12 -> Bus Creator1/8  "<overlap_f>"
  Bus Selector4/10 -> Bus Creator1/6  "<probCutIn_f>"
  Bus Selector4/11 -> Bus Creator1/7  "<probCutOut_f>"
  Bus Selector4/8 -> Vector Concatenate/4  "<probWithinLane_arr_f_3>"

== system LM_TOS_0120/LM_TOS_MODEL/adapter2/Lane_0/Subsystem5 ==
  <LANE_0_TARGETOBJECT_0_ST> : Inport
  Bus Creator1 : BusCreator  Inputs=9  OutDataTypeStr=Bus: TARGETOBJECT  NonVirtualBus=on
  Bus Selector4 : BusSelector  OutputSignals=dis2EgoLaneCenter,TTC_f,ID_un8,Index_un8,probWithinLane_arr_f_0,probWithinLane_arr_f_1,probWithinLane_arr_f_2,probWithinLane_arr_f_3,probWithinLane_arr_f_4,probCutIn_f,probCutOut_f,overlap_f,trackingTimeWithinLane_f
  Vector Concatenate : Concatenate  NumInputs=5
  TARGRTOBJECTS_ST : Outport  OutDataTypeStr=Bus: TARGETOBJECT
  wires:
  Bus Selector4/8 -> Vector Concatenate/4  "<probWithinLane_arr_f_3>"
  Bus Selector4/11 -> Bus Creator1/7  "<probCutOut_f>"
  Bus Selector4/10 -> Bus Creator1/6  "<probCutIn_f>"
  Bus Selector4/12 -> Bus Creator1/8  "<overlap_f>"
  Bus Selector4/9 -> Vector Concatenate/5  "<probWithinLane_arr_f_4>"
  Bus Selector4/2 -> Bus Creator1/2  "<TTC_f>"
  Bus Selector4/5 -> Vector Concatenate/1  "<probWithinLane_arr_f_0>"
  <LANE_0_TARGETOBJECT_0_ST>/1 -> Bus Selector4/1
  Bus Selector4/6 -> Vector Concatenate/2  "<probWithinLane_arr_f_1>"
  Bus Selector4/13 -> Bus Creator1/9  "<trackingTimeWithinLane_f>"
  Bus Selector4/1 -> Bus Creator1/1  "<dis2EgoLaneCenter>"
  Bus Selector4/7 -> Vector Concatenate/3  "<probWithinLane_arr_f_2>"
  Vector Concatenate/1 -> Bus Creator1/5
  Bus Selector4/3 -> Bus Creator1/3  "<ID_un8>"
  Bus Creator1/1 -> TARGRTOBJECTS_ST/1
  Bus Selector4/4 -> Bus Creator1/4  "<Index_un8>"

== system LM_TOS_0120/LM_TOS_MODEL/adapter2/Lane_0/Subsystem6 ==
  <LANE_0_TARGETOBJECT_0_ST> : Inport
  Bus Creator1 : BusCreator  Inputs=9  OutDataTypeStr=Bus: TARGETOBJECT  NonVirtualBus=on
  Bus Selector4 : BusSelector  OutputSignals=dis2EgoLaneCenter,TTC_f,ID_un8,Index_un8,probWithinLane_arr_f_0,probWithinLane_arr_f_1,probWithinLane_arr_f_2,probWithinLane_arr_f_3,probWithinLane_arr_f_4,probCutIn_f,probCutOut_f,overlap_f,trackingTimeWithinLane_f
  Vector Concatenate : Concatenate  NumInputs=5
  TARGRTOBJECTS_ST : Outport  OutDataTypeStr=Bus: TARGETOBJECT
  wires:
  Bus Selector4/4 -> Bus Creator1/4  "<Index_un8>"
  Bus Creator1/1 -> TARGRTOBJECTS_ST/1
  Bus Selector4/3 -> Bus Creator1/3  "<ID_un8>"
  Vector Concatenate/1 -> Bus Creator1/5
  Bus Selector4/7 -> Vector Concatenate/3  "<probWithinLane_arr_f_2>"
  Bus Selector4/1 -> Bus Creator1/1  "<dis2EgoLaneCenter>"
  Bus Selector4/13 -> Bus Creator1/9  "<trackingTimeWithinLane_f>"
  Bus Selector4/6 -> Vector Concatenate/2  "<probWithinLane_arr_f_1>"
  <LANE_0_TARGETOBJECT_0_ST>/1 -> Bus Selector4/1
  Bus Selector4/5 -> Vector Concatenate/1  "<probWithinLane_arr_f_0>"
  Bus Selector4/2 -> Bus Creator1/2  "<TTC_f>"
  Bus Selector4/9 -> Vector Concatenate/5  "<probWithinLane_arr_f_4>"
  Bus Selector4/12 -> Bus Creator1/8  "<overlap_f>"
  Bus Selector4/10 -> Bus Creator1/6  "<probCutIn_f>"
  Bus Selector4/11 -> Bus Creator1/7  "<probCutOut_f>"
  Bus Selector4/8 -> Vector Concatenate/4  "<probWithinLane_arr_f_3>"

== system LM_TOS_0120/LM_TOS_MODEL/adapter2/Lane_0/Subsystem7 ==
  <LANE_0_TARGETOBJECT_0_ST> : Inport
  Bus Creator1 : BusCreator  Inputs=9  OutDataTypeStr=Bus: TARGETOBJECT  NonVirtualBus=on
  Bus Selector4 : BusSelector  OutputSignals=dis2EgoLaneCenter,TTC_f,ID_un8,Index_un8,probWithinLane_arr_f_0,probWithinLane_arr_f_1,probWithinLane_arr_f_2,probWithinLane_arr_f_3,probWithinLane_arr_f_4,probCutIn_f,probCutOut_f,overlap_f,trackingTimeWithinLane_f
  Vector Concatenate : Concatenate  NumInputs=5
  TARGRTOBJECTS_ST : Outport  OutDataTypeStr=Bus: TARGETOBJECT
  wires:
  Bus Selector4/8 -> Vector Concatenate/4  "<probWithinLane_arr_f_3>"
  Bus Selector4/11 -> Bus Creator1/7  "<probCutOut_f>"
  Bus Selector4/10 -> Bus Creator1/6  "<probCutIn_f>"
  Bus Selector4/12 -> Bus Creator1/8  "<overlap_f>"
  Bus Selector4/9 -> Vector Concatenate/5  "<probWithinLane_arr_f_4>"
  Bus Selector4/2 -> Bus Creator1/2  "<TTC_f>"
  Bus Selector4/5 -> Vector Concatenate/1  "<probWithinLane_arr_f_0>"
  <LANE_0_TARGETOBJECT_0_ST>/1 -> Bus Selector4/1
  Bus Selector4/6 -> Vector Concatenate/2  "<probWithinLane_arr_f_1>"
  Bus Selector4/13 -> Bus Creator1/9  "<trackingTimeWithinLane_f>"
  Bus Selector4/1 -> Bus Creator1/1  "<dis2EgoLaneCenter>"
  Bus Selector4/7 -> Vector Concatenate/3  "<probWithinLane_arr_f_2>"
  Vector Concatenate/1 -> Bus Creator1/5
  Bus Selector4/3 -> Bus Creator1/3  "<ID_un8>"
  Bus Creator1/1 -> TARGRTOBJECTS_ST/1
  Bus Selector4/4 -> Bus Creator1/4  "<Index_un8>"

== system LM_TOS_0120/LM_TOS_MODEL/adapter2/Lane_0/Subsystem8 ==
  <LANE_0_TARGETOBJECT_0_ST> : Inport
  Bus Creator1 : BusCreator  Inputs=9  OutDataTypeStr=Bus: TARGETOBJECT  NonVirtualBus=on
  Bus Selector4 : BusSelector  OutputSignals=dis2EgoLaneCenter,TTC_f,ID_un8,Index_un8,probWithinLane_arr_f_0,probWithinLane_arr_f_1,probWithinLane_arr_f_2,probWithinLane_arr_f_3,probWithinLane_arr_f_4,probCutIn_f,probCutOut_f,overlap_f,trackingTimeWithinLane_f
  Vector Concatenate : Concatenate  NumInputs=5
  TARGRTOBJECTS_ST : Outport  OutDataTypeStr=Bus: TARGETOBJECT
  wires:
  Bus Selector4/4 -> Bus Creator1/4  "<Index_un8>"
  Bus Creator1/1 -> TARGRTOBJECTS_ST/1
  Bus Selector4/3 -> Bus Creator1/3  "<ID_un8>"
  Vector Concatenate/1 -> Bus Creator1/5
  Bus Selector4/7 -> Vector Concatenate/3  "<probWithinLane_arr_f_2>"
  Bus Selector4/1 -> Bus Creator1/1  "<dis2EgoLaneCenter>"
  Bus Selector4/13 -> Bus Creator1/9  "<trackingTimeWithinLane_f>"
  Bus Selector4/6 -> Vector Concatenate/2  "<probWithinLane_arr_f_1>"
  <LANE_0_TARGETOBJECT_0_ST>/1 -> Bus Selector4/1
  Bus Selector4/5 -> Vector Concatenate/1  "<probWithinLane_arr_f_0>"
  Bus Selector4/2 -> Bus Creator1/2  "<TTC_f>"
  Bus Selector4/9 -> Vector Concatenate/5  "<probWithinLane_arr_f_4>"
  Bus Selector4/12 -> Bus Creator1/8  "<overlap_f>"
  Bus Selector4/10 -> Bus Creator1/6  "<probCutIn_f>"
  Bus Selector4/11 -> Bus Creator1/7  "<probCutOut_f>"
  Bus Selector4/8 -> Vector Concatenate/4  "<probWithinLane_arr_f_3>"

== system LM_TOS_0120/LM_TOS_MODEL/adapter2/Lane_0/Subsystem9 ==
  <LANE_0_TARGETOBJECT_0_ST> : Inport
  Bus Creator1 : BusCreator  Inputs=9  OutDataTypeStr=Bus: TARGETOBJECT  NonVirtualBus=on
  Bus Selector4 : BusSelector  OutputSignals=dis2EgoLaneCenter,TTC_f,ID_un8,Index_un8,probWithinLane_arr_f_0,probWithinLane_arr_f_1,probWithinLane_arr_f_2,probWithinLane_arr_f_3,probWithinLane_arr_f_4,probCutIn_f,probCutOut_f,overlap_f,trackingTimeWithinLane_f
  Vector Concatenate : Concatenate  NumInputs=5
  TARGRTOBJECTS_ST : Outport  OutDataTypeStr=Bus: TARGETOBJECT
  wires:
  Bus Selector4/8 -> Vector Concatenate/4  "<probWithinLane_arr_f_3>"
  Bus Selector4/11 -> Bus Creator1/7  "<probCutOut_f>"
  Bus Selector4/10 -> Bus Creator1/6  "<probCutIn_f>"
  Bus Selector4/12 -> Bus Creator1/8  "<overlap_f>"
  Bus Selector4/9 -> Vector Concatenate/5  "<probWithinLane_arr_f_4>"
  Bus Selector4/2 -> Bus Creator1/2  "<TTC_f>"
  Bus Selector4/5 -> Vector Concatenate/1  "<probWithinLane_arr_f_0>"
  <LANE_0_TARGETOBJECT_0_ST>/1 -> Bus Selector4/1
  Bus Selector4/6 -> Vector Concatenate/2  "<probWithinLane_arr_f_1>"
  Bus Selector4/13 -> Bus Creator1/9  "<trackingTimeWithinLane_f>"
  Bus Selector4/1 -> Bus Creator1/1  "<dis2EgoLaneCenter>"
  Bus Selector4/7 -> Vector Concatenate/3  "<probWithinLane_arr_f_2>"
  Vector Concatenate/1 -> Bus Creator1/5
  Bus Selector4/3 -> Bus Creator1/3  "<ID_un8>"
  Bus Creator1/1 -> TARGRTOBJECTS_ST/1
  Bus Selector4/4 -> Bus Creator1/4  "<Index_un8>"

== system LM_TOS_0120/LM_TOS_MODEL/adapter2/Lane_1/Subsystem ==
  <LANE_1_TARGETOBJECT_0_ST> : Inport
  Bus Creator1 : BusCreator  Inputs=9  OutDataTypeStr=Bus: TARGETOBJECT  NonVirtualBus=on
  Bus Selector4 : BusSelector  OutputSignals=dis2EgoLaneCenter,TTC_f,ID_un8,Index_un8,probWithinLane_arr_f_0,probWithinLane_arr_f_1,probWithinLane_arr_f_2,probWithinLane_arr_f_3,probWithinLane_arr_f_4,probCutIn_f,probCutOut_f,overlap_f,trackingTimeWithinLane_f
  Vector Concatenate : Concatenate  NumInputs=5
  TARGRTOBJECTS_ST : Outport  OutDataTypeStr=Bus: TARGETOBJECT
  wires:
  Bus Selector4/8 -> Vector Concatenate/4  "<probWithinLane_arr_f_3>"
  Bus Selector4/11 -> Bus Creator1/7  "<probCutOut_f>"
  Bus Selector4/10 -> Bus Creator1/6  "<probCutIn_f>"
  Bus Selector4/12 -> Bus Creator1/8  "<overlap_f>"
  Bus Selector4/9 -> Vector Concatenate/5  "<probWithinLane_arr_f_4>"
  Bus Selector4/2 -> Bus Creator1/2  "<TTC_f>"
  Bus Selector4/5 -> Vector Concatenate/1  "<probWithinLane_arr_f_0>"
  <LANE_1_TARGETOBJECT_0_ST>/1 -> Bus Selector4/1
  Bus Selector4/6 -> Vector Concatenate/2  "<probWithinLane_arr_f_1>"
  Bus Selector4/13 -> Bus Creator1/9  "<trackingTimeWithinLane_f>"
  Bus Selector4/1 -> Bus Creator1/1  "<dis2EgoLaneCenter>"
  Bus Selector4/7 -> Vector Concatenate/3  "<probWithinLane_arr_f_2>"
  Vector Concatenate/1 -> Bus Creator1/5
  Bus Selector4/3 -> Bus Creator1/3  "<ID_un8>"
  Bus Creator1/1 -> TARGRTOBJECTS_ST/1
  Bus Selector4/4 -> Bus Creator1/4  "<Index_un8>"

== system LM_TOS_0120/LM_TOS_MODEL/adapter2/Lane_1/Subsystem1 ==
  <LANE_1_TARGETOBJECT_0_ST> : Inport
  Bus Creator1 : BusCreator  Inputs=9  OutDataTypeStr=Bus: TARGETOBJECT  NonVirtualBus=on
  Bus Selector4 : BusSelector  OutputSignals=dis2EgoLaneCenter,TTC_f,ID_un8,Index_un8,probWithinLane_arr_f_0,probWithinLane_arr_f_1,probWithinLane_arr_f_2,probWithinLane_arr_f_3,probWithinLane_arr_f_4,probCutIn_f,probCutOut_f,overlap_f,trackingTimeWithinLane_f
  Vector Concatenate : Concatenate  NumInputs=5
  TARGRTOBJECTS_ST : Outport  OutDataTypeStr=Bus: TARGETOBJECT
  wires:
  Bus Selector4/4 -> Bus Creator1/4  "<Index_un8>"
  Bus Creator1/1 -> TARGRTOBJECTS_ST/1
  Bus Selector4/3 -> Bus Creator1/3  "<ID_un8>"
  Vector Concatenate/1 -> Bus Creator1/5
  Bus Selector4/7 -> Vector Concatenate/3  "<probWithinLane_arr_f_2>"
  Bus Selector4/1 -> Bus Creator1/1  "<dis2EgoLaneCenter>"
  Bus Selector4/13 -> Bus Creator1/9  "<trackingTimeWithinLane_f>"
  Bus Selector4/6 -> Vector Concatenate/2  "<probWithinLane_arr_f_1>"
  <LANE_1_TARGETOBJECT_0_ST>/1 -> Bus Selector4/1
  Bus Selector4/5 -> Vector Concatenate/1  "<probWithinLane_arr_f_0>"
  Bus Selector4/2 -> Bus Creator1/2  "<TTC_f>"
  Bus Selector4/9 -> Vector Concatenate/5  "<probWithinLane_arr_f_4>"
  Bus Selector4/12 -> Bus Creator1/8  "<overlap_f>"
  Bus Selector4/10 -> Bus Creator1/6  "<probCutIn_f>"
  Bus Selector4/11 -> Bus Creator1/7  "<probCutOut_f>"
  Bus Selector4/8 -> Vector Concatenate/4  "<probWithinLane_arr_f_3>"

== system LM_TOS_0120/LM_TOS_MODEL/adapter2/Lane_1/Subsystem10 ==
  <LANE_1_TARGETOBJECT_0_ST> : Inport
  Bus Creator1 : BusCreator  Inputs=7  OutDataTypeStr=Bus: SEGMENT  NonVirtualBus=on
  Bus Selector4 : BusSelector  OutputSignals=coef_arr_f_0,coef_arr_f_1,coef_arr_f_2,coef_arr_f_3,dlowerLimit_f,dupperLimit_f,numOfSegment_un8,available_b,detectedByVideo_b,quality_f
  Vector Concatenate : Concatenate  NumInputs=4
  SEGMENT_ST : Outport  OutDataTypeStr=Bus: SEGMENT
  wires:
  Bus Selector4/6 -> Bus Creator1/3  "<dupperLimit_f>"
  Bus Selector4/7 -> Bus Creator1/4  "<numOfSegment_un8>"
  Bus Selector4/8 -> Bus Creator1/5  "<available_b>"
  Bus Selector4/9 -> Bus Creator1/6  "<detectedByVideo_b>"
  Bus Selector4/10 -> Bus Creator1/7  "<quality_f>"
  Bus Selector4/5 -> Bus Creator1/2  "<dlowerLimit_f>"
  Vector Concatenate/1 -> Bus Creator1/1
  Bus Selector4/4 -> Vector Concatenate/4  "<coef_arr_f_3>"
  Bus Selector4/3 -> Vector Concatenate/3  "<coef_arr_f_2>"
  Bus Selector4/1 -> Vector Concatenate/1  "<coef_arr_f_0>"
  Bus Selector4/2 -> Vector Concatenate/2  "<coef_arr_f_1>"
  <LANE_1_TARGETOBJECT_0_ST>/1 -> Bus Selector4/1
  Bus Creator1/1 -> SEGMENT_ST/1

== system LM_TOS_0120/LM_TOS_MODEL/adapter2/Lane_1/Subsystem11 ==
  <LANE_1_TARGETOBJECT_0_ST> : Inport
  Bus Creator1 : BusCreator  Inputs=7  OutDataTypeStr=Bus: SEGMENT  NonVirtualBus=on
  Bus Selector4 : BusSelector  OutputSignals=coef_arr_f_0,coef_arr_f_1,coef_arr_f_2,coef_arr_f_3,dlowerLimit_f,dupperLimit_f,numOfSegment_un8,available_b,detectedByVideo_b,quality_f
  Vector Concatenate : Concatenate  NumInputs=4
  SEGMENT_ST : Outport  OutDataTypeStr=Bus: SEGMENT
  wires:
  Bus Creator1/1 -> SEGMENT_ST/1
  <LANE_1_TARGETOBJECT_0_ST>/1 -> Bus Selector4/1
  Bus Selector4/2 -> Vector Concatenate/2  "<coef_arr_f_1>"
  Bus Selector4/1 -> Vector Concatenate/1  "<coef_arr_f_0>"
  Bus Selector4/3 -> Vector Concatenate/3  "<coef_arr_f_2>"
  Bus Selector4/4 -> Vector Concatenate/4  "<coef_arr_f_3>"
  Vector Concatenate/1 -> Bus Creator1/1
  Bus Selector4/5 -> Bus Creator1/2  "<dlowerLimit_f>"
  Bus Selector4/10 -> Bus Creator1/7  "<quality_f>"
  Bus Selector4/9 -> Bus Creator1/6  "<detectedByVideo_b>"
  Bus Selector4/8 -> Bus Creator1/5  "<available_b>"
  Bus Selector4/7 -> Bus Creator1/4  "<numOfSegment_un8>"
  Bus Selector4/6 -> Bus Creator1/3  "<dupperLimit_f>"

== system LM_TOS_0120/LM_TOS_MODEL/adapter2/Lane_1/Subsystem12 ==
  <LANE_1_TARGETOBJECT_0_ST> : Inport
  Bus Creator1 : BusCreator  Inputs=7  OutDataTypeStr=Bus: SEGMENT  NonVirtualBus=on
  Bus Selector4 : BusSelector  OutputSignals=coef_arr_f_0,coef_arr_f_1,coef_arr_f_2,coef_arr_f_3,dlowerLimit_f,dupperLimit_f,numOfSegment_un8,available_b,detectedByVideo_b,quality_f
  Vector Concatenate : Concatenate  NumInputs=4
  SEGMENT_ST : Outport  OutDataTypeStr=Bus: SEGMENT
  wires:
  Bus Selector4/6 -> Bus Creator1/3  "<dupperLimit_f>"
  Bus Selector4/7 -> Bus Creator1/4  "<numOfSegment_un8>"
  Bus Selector4/8 -> Bus Creator1/5  "<available_b>"
  Bus Selector4/9 -> Bus Creator1/6  "<detectedByVideo_b>"
  Bus Selector4/10 -> Bus Creator1/7  "<quality_f>"
  Bus Selector4/5 -> Bus Creator1/2  "<dlowerLimit_f>"
  Vector Concatenate/1 -> Bus Creator1/1
  Bus Selector4/4 -> Vector Concatenate/4  "<coef_arr_f_3>"
  Bus Selector4/3 -> Vector Concatenate/3  "<coef_arr_f_2>"
  Bus Selector4/1 -> Vector Concatenate/1  "<coef_arr_f_0>"
  Bus Selector4/2 -> Vector Concatenate/2  "<coef_arr_f_1>"
  <LANE_1_TARGETOBJECT_0_ST>/1 -> Bus Selector4/1
  Bus Creator1/1 -> SEGMENT_ST/1
